simulink model "Limiter"  (R2022b)
settings: Solver=VariableStepAuto  StartTime=0.0  StopTime=10.0  RelTol=1e-3
settings Model: Creator=mliu  LastModifiedBy=mliu

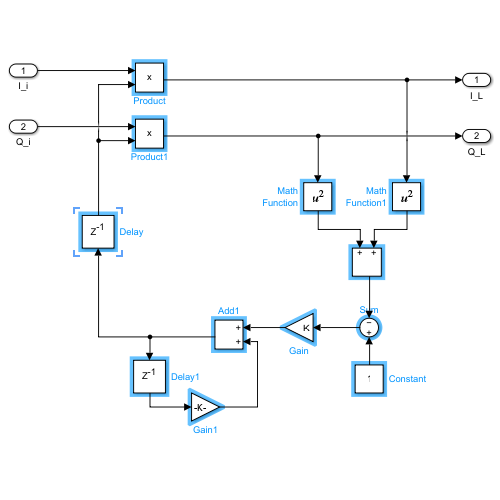
[thumbnail: Simulink's stored preview of the top-level diagram]
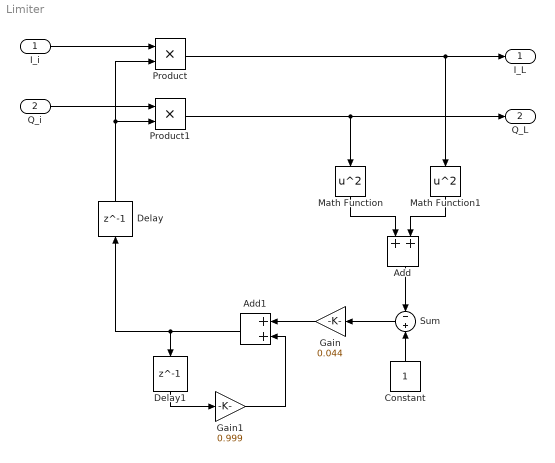
== system Limiter ==
  I_i : Inport
  Q_i : Inport  Port=2
  Add : Sum
  Add1 : Sum
  Constant : Constant
  Delay : Delay  DelayLength=1  InitialCondition=0
  Delay1 : Delay  DelayLength=1  InitialCondition=0
  Gain : Gain  Gain=0.044
  Gain1 : Gain  Gain=0.999
  Math Function : Math  Operator=square
  Math Function1 : Math  Operator=square
  Product : Product
  Product1 : Product
  Sum : Sum  Inputs=-|+
  I_L : Outport
  Q_L : Outport  Port=2
  wires:
  Product/1 -> Math Function1/1, I_L/1
  Product1/1 -> Math Function/1, Q_L/1
  I_i/1 -> Product/1
  Q_i/1 -> Product1/1
  Math Function1/1 -> Add/2
  Math Function/1 -> Add/1
  Add/1 -> Sum/1
  Constant/1 -> Sum/2
  Delay/1 -> Product1/2, Product/2
  Sum/1 -> Gain/1
  Gain/1 -> Add1/1
  Add1/1 -> Delay1/1, Delay/1
  Delay1/1 -> Gain1/1
  Gain1/1 -> Add1/2
